simulink model "project"  (R2022b)
settings: Solver=VariableStepAuto  StartTime=0.0  StopTime=simulation_time  RelTol=1e-3
values from neighbouring files (symbols this model uses):
  sampling_time = Ts    (= 0.001)    [main.m]
settings Model: Creator=jernej sabadin  LastModifiedBy=jernej sabadin

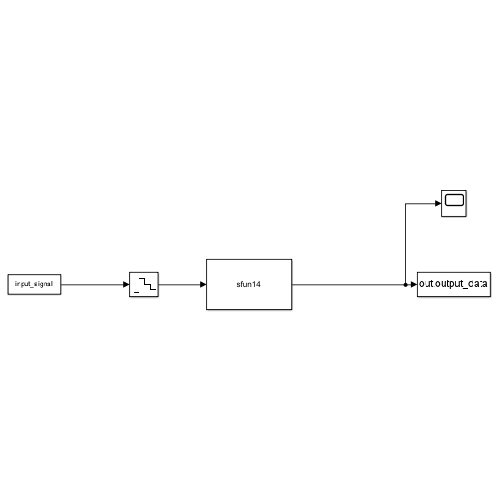
[thumbnail: Simulink's stored preview of the top-level diagram]
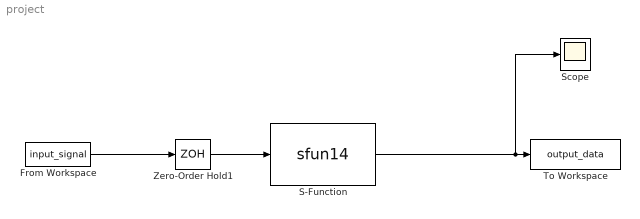
== system project ==
  From Workspace : FromWorkspace  VariableName=input_signal  SampleTime=sampling_time
  S-Function : S-Function  FunctionName=sfun14  SFunctionDeploymentMode=off  EnableBusSupport=off
  Scope : Scope
  To Workspace : ToWorkspace  VariableName=output_data  SaveFormat=Timeseries  SampleTime=sampling_time
  Zero-Order Hold1 : ZeroOrderHold  SampleTime=sampling_time
  wires:
  From Workspace/1 -> Zero-Order Hold1/1
  S-Function/1 -> Scope/1, To Workspace/1
  Zero-Order Hold1/1 -> S-Function/1
